simulink model "simulation_lqr"  (R2020b)
settings: Solver=VariableStepAuto  StartTime=0.0  StopTime=10  RelTol=1e-3
values from neighbouring files (symbols this model uses):
  K_lqr = lqr(A,B,Q_lqr,R_lqr)    [make_lqr.m]
undefined symbols (not defined in the file or in its folder): qe, ue
settings Model: Creator=block  LastModifiedBy=block

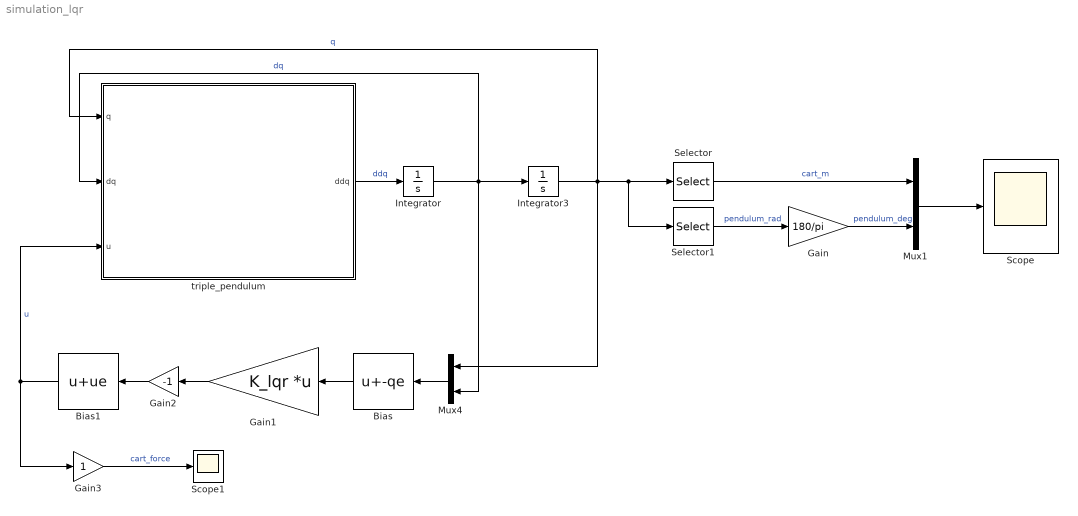
== system simulation_lqr ==
  Bias : Bias  Bias=-qe
  Bias1 : Bias  Bias=ue
  Gain : Gain  Gain=180/pi
  Gain1 : Gain  Gain=K_lqr  Multiplication=Matrix(K*u)
  Gain2 : Gain  Gain=-1
  Gain3 : Gain
  Integrator : Integrator  InitialCondition=[0;0;0;0]
  Integrator3 : Integrator  InitialCondition=[0;pi*5/180;0;0]
  Mux1 : Mux  Inputs=2
  Mux4 : Mux  Inputs=2
  Scope : Scope
  Scope1 : Scope
  Selector : Selector  InputPortWidth=4  IndexOptions=Index vector (dialog)  Indices=1  OutputSizes=1
  Selector1 : Selector  InputPortWidth=4  IndexOptions=Index vector (dialog)  Indices=[2,3,4]  OutputSizes=1
  triple_pendulum : MATLAB Function  TreatAsAtomicUnit=on
  wires:
  Gain1/1 -> Gain2/1
  Mux4/1 -> Bias/1
  Integrator/1 -> Integrator3/1, triple_pendulum/2(dq), Mux4/2  "dq"
  Gain2/1 -> Bias1/1
  triple_pendulum/1(ddq) -> Integrator/1  "ddq"
  Bias/1 -> Gain1/1
  Bias1/1 -> triple_pendulum/3(u), Gain3/1  "u"
  Integrator3/1 -> Selector1/1, Selector/1, Mux4/1, triple_pendulum/1(q)  "q"
  Selector/1 -> Mux1/1  "cart_m"
  Gain/1 -> Mux1/2  "pendulum_deg"
  Mux1/1 -> Scope/1
  Selector1/1 -> Gain/1  "pendulum_rad"
  Gain3/1 -> Scope1/1  "cart_force"

== matlab function simulation_lqr/triple_pendulum ==
  data: q input; ddq output; dq input; u input
function ddq = triple_pendulum(q,dq,u)
    ddq = ode(q(1),q(2),q(3),q(4),dq(1),dq(2),dq(3),dq(4),u(1),0,0,0);
end
